simulink model "TRIAD_testbench"  (R2025b)
settings: Solver=VariableStepAuto  StartTime=0.0  StopTime=90*60  RelTol=1e-3
undefined symbols (not defined in the file or in its folder): WMM2025
libraries: aerolibutil x4, dspmathops x4, aerolibtransform2 x1, sharedutil x1, matrix_library x1, aerolibgravity2 x1
settings Model: Creator=chass  LastModifiedBy=chass

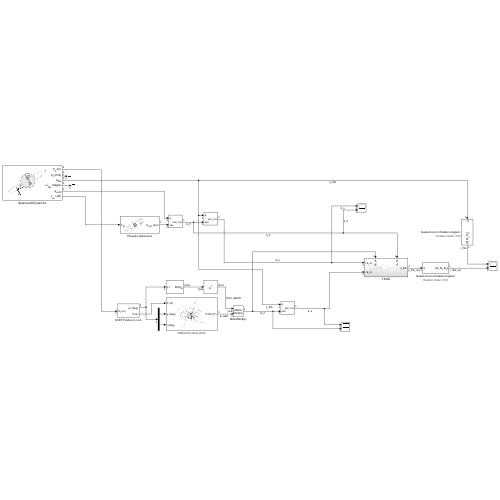
[thumbnail: Simulink's stored preview of the top-level diagram]
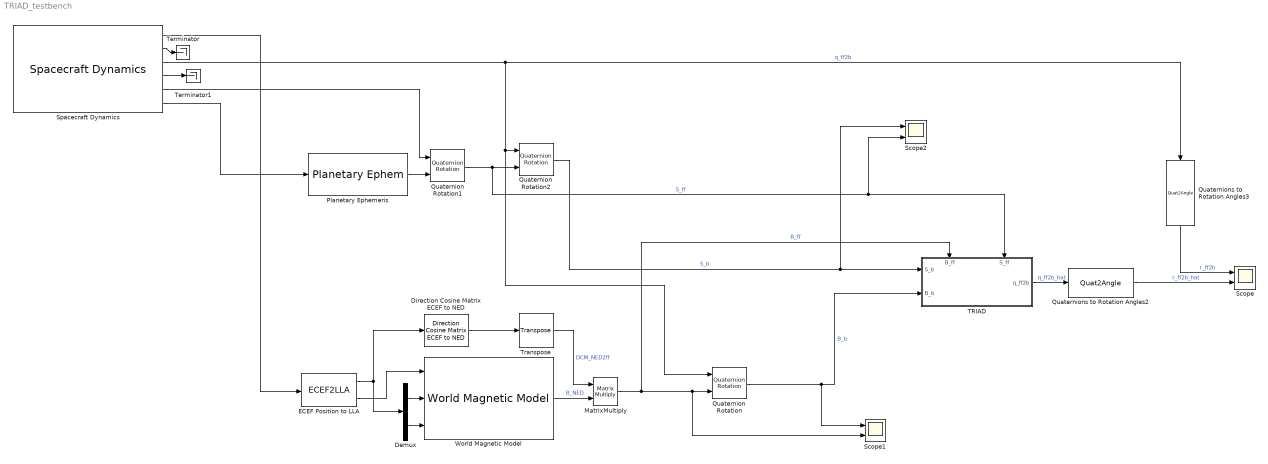
== system TRIAD_testbench ==
  Demux : Demux  Outputs=2
  Direction Cosine Matrix ECEF to NED : aerolibtransform2/Direction Cosine Matrix ECEF to NED
  ECEF Position to LLA : ECEF2LLA
  MatrixMultiply : Product  Multiplication=Matrix(*)
  Planetary Ephemeris : PlanetaryEphem  target=Sun  outputVelocity=off
  Quaternion Rotation : aerolibutil/Quaternion Rotation
  Quaternion Rotation1 : aerolibutil/Quaternion Rotation
  Quaternion Rotation2 : aerolibutil/Quaternion Rotation
  Quaternions to Rotation Angles2 : Quat2Angle  rotationOrder=XYZ
      settings: AttributesFormatString=Rotation Order: %<rotationOrder>
  Quaternions to Rotation Angles3 : Quat2Angle  rotationOrder=XYZ
      settings: AttributesFormatString=Rotation Order: %<rotationOrder>
  Scope : Scope  NumInputPorts=2
      settings: ActiveDisplayYMinimum=-4.0237003189636624  ActiveDisplayYMaximum=2.3753171663449577
  Scope1 : Scope  NumInputPorts=2
      settings: ActiveDisplayYMinimum=-90706.468158005373  ActiveDisplayYMaximum=49109.361957621222
  Scope2 : Scope  NumInputPorts=2
      settings: ActiveDisplayYMinimum=-1.3526055933478013E+8  ActiveDisplayYMaximum=1.7791445102441102E+8  DataLoggingVariableName=ScopeData2
  Spacecraft Dynamics : SpacecraftDynamics  forcesIn=off  momentsIn=off  outportFrame=Fixed-frame  attitudeFrame=Fixed-frame  attitudeRate=[1, 0, 0]  outputTransform=on
  TRIAD : Subsystem
      settings: PortSchema="{\"entries\":[{\"content\":{\"sides\":[{\"content\":{\"connectorIds\":[\"In1\",\"In2\"]},\"type\":\"ConnectorPlacement.EquallySpacedRectSide\",\"uuid\":\"934d396e-f242-4144-8e49-7dca4c529b1e\"},{\"content\":{\"connectorIds\":[\"Out1\"],\"side\":\"RIGHT\"},\"type\":\"ConnectorPlacement.EquallySpacedRectSide\",\"uuid\":\"d5049cd6-8da5-467a-a595-0659620b3453\"},{\"content\":{\"connectorIds\":[\"In3\",\"In4\"],\"side\":\"TOP\"},\"type\":\"ConnectorPlacement.EquallySpacedRectSide\",\"uuid\":\"566a2326-4576-4247-b03e-f5181e2b65c9\"}]},\"type\":\"ConnectorPlacement.EquallySpacedConnector\",\"uuid\":\"3190049e-3c9f-4103-9960-cf9fc3914e67\"}],\"packageUris\":[\"http://schema.mathworks.com/mf0/Connector/R2020b\"],\"version\":\"1.0\"}"
  Terminator : Terminator
  Terminator1 : Terminator
  Transpose : matrix_library/Transpose
  World Magnetic Model : aerolibgravity2/World Magnetic Model  model=WMM2025 (2025-2030)  customFile='WMM2025.COF'  units=Metric (MKS)  time_in=off  month=January  day=1  year=2025  action=Error  h_out=off  dec_out=off  inc_out=off  ti_out=off
  wires:
  Spacecraft Dynamics/2 -> Terminator/1
  Spacecraft Dynamics/3 -> Quaternion Rotation/1, Quaternion Rotation2/1, Quaternions to Rotation Angles3/1  "q_ff2b"
  Spacecraft Dynamics/6 -> Planetary Ephemeris/1
  Spacecraft Dynamics/1 -> ECEF Position to LLA/1
  Quaternion Rotation2/1 -> Scope2/1, TRIAD/1(S_b)  "S_b"
  ECEF Position to LLA/2 -> World Magnetic Model/1
  Demux/1 -> World Magnetic Model/2
  Demux/2 -> World Magnetic Model/3
  ECEF Position to LLA/1 -> Demux/1, Direction Cosine Matrix ECEF to NED/1
  Direction Cosine Matrix ECEF to NED/1 -> Transpose/1
  World Magnetic Model/1 -> MatrixMultiply/2  "B_NED"
  Transpose/1 -> MatrixMultiply/1  "DCM_NED2ff"
  MatrixMultiply/1 -> TRIAD/3(B_ff), Scope1/2, Quaternion Rotation/2  "B_ff"
  Quaternion Rotation/1 -> Scope1/1, TRIAD/2(B_b)  "B_b"
  Quaternion Rotation1/1 -> Quaternion Rotation2/2, Scope2/2, TRIAD/4(S_ff)  "S_ff"
  TRIAD/1(q_ff2b) -> Quaternions to Rotation Angles2/1  "q_ff2b_hat"
  Quaternions to Rotation Angles2/1 -> Scope/2  "r_ff2b_hat"
  Quaternions to Rotation Angles3/1 -> Scope/1  "r_ff2b"
  Spacecraft Dynamics/4 -> Terminator1/1
  Planetary Ephemeris/1 -> Quaternion Rotation1/2
  Spacecraft Dynamics/5 -> Quaternion Rotation1/1

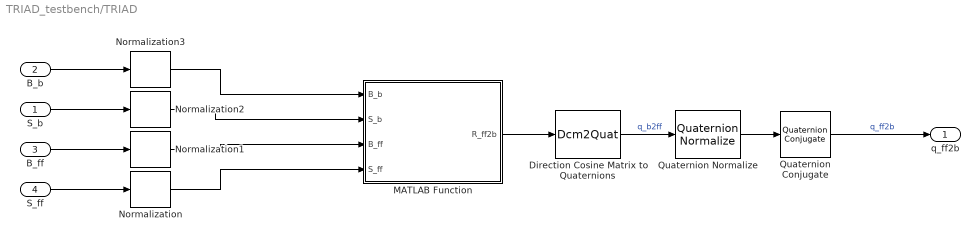
== system TRIAD_testbench/TRIAD ==
  S_b : Inport
  B_b : Inport  Port=2
  B_ff : Inport  Port=3
  S_ff : Inport  Port=4
  Direction Cosine Matrix to Quaternions : Dcm2Quat
  MATLAB Function : MATLAB Function  TreatAsAtomicUnit=on
  Normalization{,1..3} (4 alike) : dspmathops/Normalization  NormType=2-norm  Bias=0  NormOver=Each column  Dimension=1  roundingMode=Floor  overflowMode=off  accumDataTypeStr=Inherit: Same as product output  accumLastDataTypeStr=Inherit: Same as product output  outputDataTypeStr=Inherit: Same as product output  outputMin=[]  outputMax=[]  outputLastDataTypeStr=Inherit: Same as product output
  Quaternion Conjugate : aerolibutil/Quaternion Conjugate
  Quaternion Normalize : sharedutil/Quaternion Normalize  aMode=aMode
  q_ff2b : Outport
  wires:
  B_ff/1 -> Normalization1/1
  S_ff/1 -> Normalization/1
  MATLAB Function/1(R_ff2b) -> Direction Cosine Matrix to Quaternions/1
  Direction Cosine Matrix to Quaternions/1 -> Quaternion Normalize/1  "q_b2ff"
  Quaternion Normalize/1 -> Quaternion Conjugate/1
  B_b/1 -> Normalization3/1
  S_b/1 -> Normalization2/1
  Normalization3/1 -> MATLAB Function/1(B_b)
  Normalization2/1 -> MATLAB Function/2(S_b)
  Normalization1/1 -> MATLAB Function/3(B_ff)
  Normalization/1 -> MATLAB Function/4(S_ff)
  Quaternion Conjugate/1 -> q_ff2b/1  "q_ff2b"

== matlab function TRIAD_testbench/TRIAD/MATLAB Function ==
  data: B_b input; R_ff2b output; S_b input; B_ff input; S_ff input
function R_ff2b = TRIAD1(B_b, S_b, B_ff, S_ff)






t1_b = S_b;
t2_b = cross(S_b, B_b)/norm(cross(S_b, B_b));
t3_b = cross(t1_b, t2_b);

t1_f = S_ff;
t2_f = cross(S_ff, B_ff)/norm(cross(S_ff, B_ff));
t3_f = cross(t1_f, t2_f);

R_bt = [t1_b t2_b t3_b];
R_ft = [t1_f t2_f t3_f];

R_bf = R_bt*R_ft';

R_ff2b = R_bf';
